simulink model "BE3_auto"  (R2018b)
settings: Solver=VariableStepAuto  StartTime=0.0  StopTime=50  RelTol=1e-3
values from neighbouring files (symbols this model uses):
  A = [1  a1 a2]    [BE2_auto.m]    (also in BE6_7et8_auto.m = [l1 0 0; 0 0 1; l2 l3 0]; BE_synthese.m = [-alpha1 0; alpha1 -alpha2])
  B = [0 b1 b2]    [BE2_auto.m]    (also in BE6_7et8_auto.m = [l4; 0; 0]; BE_synthese.m = [sigma0; 0])
  R = [r0 r1 r2]    [BE2_auto.m]    (also in BE6_7et8_auto.m = 1; BE_synthese.m)
  S = [1 (sp1-1) -sp1]    [BE2_auto.m]    (also in BE_synthese.m)
settings Model: Creator=piffercg  LastModifiedBy=piffercg

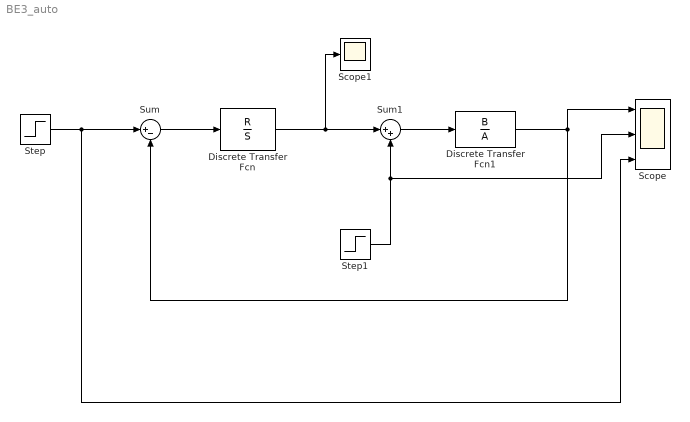
== system BE3_auto ==
  Discrete Transfer Fcn : DiscreteTransferFcn  Numerator=R  Denominator=S  SampleTime=1
  Discrete Transfer Fcn1 : DiscreteTransferFcn  Numerator=B  Denominator=A  SampleTime=1
  Scope : Scope  NumInputPorts=3
  Scope1 : Scope
  Step : Step  SampleTime=0
  Step1 : Step  Time=20  After=-1  SampleTime=0
  Sum : Sum  Inputs=|+-
  Sum1 : Sum  Inputs=|++
  wires:
  Step/1 -> Scope/3, Sum/1
  Sum/1 -> Discrete Transfer Fcn/1
  Discrete Transfer Fcn/1 -> Scope1/1, Sum1/1
  Sum1/1 -> Discrete Transfer Fcn1/1
  Discrete Transfer Fcn1/1 -> Sum/2, Scope/1
  Step1/1 -> Scope/2, Sum1/2
